simulink model "am_ssb_moding_sine_signal"  (R2022b)
settings: Solver=VariableStepAuto  StartTime=0.0  StopTime=0.06  RelTol=1e-3
undefined symbols (not defined in the file or in its folder): fdesignblkfcn, gcbh
libraries: dspsrcs4 x6
settings Model: Creator=kalyan  LastModifiedBy=kalyan

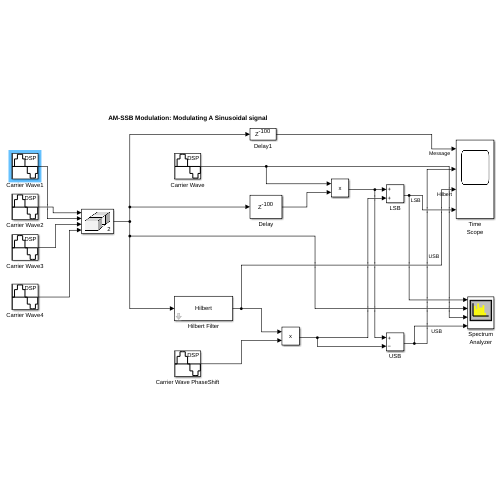
[thumbnail: Simulink's stored preview of the top-level diagram]
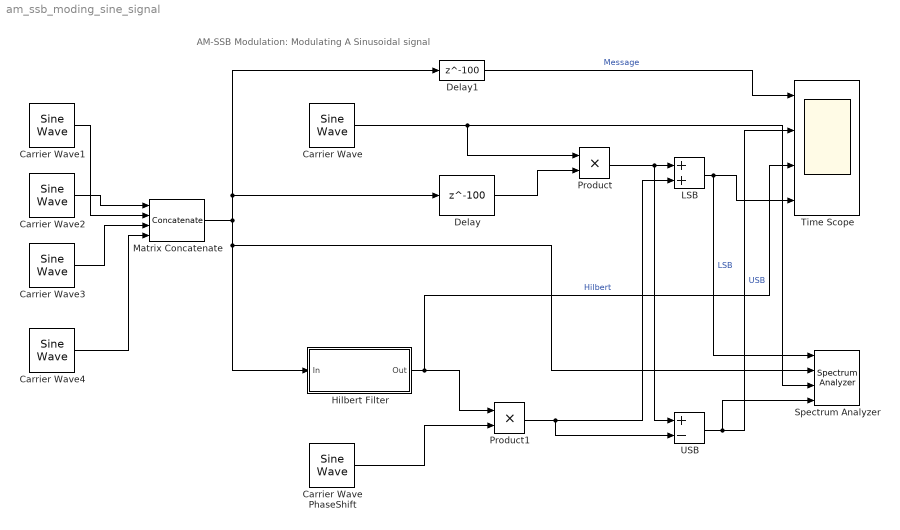
== system am_ssb_moding_sine_signal ==
  note: AM-SSB Modulation: Modulating A Sinusoidal signal
  Carrier Wave{,1..4} (5 alike) : dspsrcs4/Sine Wave  Amplitude=3  Frequency=15000  Phase=1.5708  SampleMode=Discrete  OutComplex=Real  CompMethod=Trigonometric fcn  TableSize=Speed  SampleTime=1/200000  SamplesPerFrame=1  ResetState=Restart at time zero  OutputFrames=off  dataType=double  wordLen=16  udDataType=sfix(16)  fracBitsMode=Best precision  numFracBits=15  OutDataTypeStr=double  LastOutDataTypeStr=double
  Carrier Wave PhaseShift : dspsrcs4/Sine Wave  Amplitude=3  Frequency=15000  Phase=1.5708 - (pi/2)  SampleMode=Discrete  OutComplex=Real  CompMethod=Trigonometric fcn  TableSize=Speed  SampleTime=1/200000  SamplesPerFrame=1  ResetState=Restart at time zero  OutputFrames=off  dataType=double  wordLen=16  udDataType=sfix(16)  fracBitsMode=Best precision  numFracBits=15  OutDataTypeStr=double  LastOutDataTypeStr=double
  Delay : Delay  DelayLength=100  InitialCondition=0  UseCircularBuffer=on
  Delay1 : Delay  DelayLength=100  InitialCondition=0  UseCircularBuffer=on
  Hilbert Filter : Subsystem  DialogController=fdesignblkfcn  InitFcn=fdesignblkfcn(gcbh, {'InitFcn'});  mask(Hilbert Filter){}
      mask help: Design a Hilbert filter
      settings: CopyFcn=fdesignblkfcn(gcbh, {'CopyFcn'});
      mask Help: helpview(mapfilelocation('dsp'), 'dsphilbertfilter');
      mask Display: disp('Hilbert')
  LSB : Sum
  Matrix Concatenate : Concatenate  NumInputs=4  Mode=Multidimensional array  ConcatenateDimension=2
  Product : Product
  Product1 : Product
  Spectrum Analyzer : SpectrumAnalyzer  NumInputPorts=4
  Time Scope : Scope  NumInputPorts=4
  USB : Sum  Inputs=+-
  wires:
  Matrix Concatenate/1 -> Spectrum Analyzer/2, Hilbert Filter/1(In), Delay1/1, Delay/1
  Delay/1 -> Product/2
  Carrier Wave/1 -> Spectrum Analyzer/3, Product/1
  Carrier Wave PhaseShift/1 -> Product1/2
  Hilbert Filter/1(Out) -> Time Scope/3, Product1/1  "Hilbert"
  Product/1 -> USB/1, LSB/1
  Product1/1 -> USB/2, LSB/2
  LSB/1 -> Spectrum Analyzer/1, Time Scope/4  "LSB"
  USB/1 -> Spectrum Analyzer/4, Time Scope/2  "USB"
  Delay1/1 -> Time Scope/1  "Message"
  Carrier Wave1/1 -> Matrix Concatenate/2
  Carrier Wave2/1 -> Matrix Concatenate/1
  Carrier Wave3/1 -> Matrix Concatenate/3
  Carrier Wave4/1 -> Matrix Concatenate/4

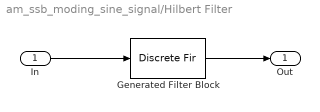
== system am_ssb_moding_sine_signal/Hilbert Filter ==
  In : Inport
  Generated Filter Block : DiscreteFir  Tag=BlockMethodSubSystem  Coefficients=[5.15003860718366009e-16 -8.3766156093727947e-05 2.35802139276509804e-15 -6.59921120241440854e-05 -6.21131926040260173e-16 -9.1525954819813264e-05 -2.00176151456124911e-15 -0.000123132434560440258 -3.05107280552708726e-16 -0.000161730665024954116 1.75952430435556519e-16 -0.000208423670586796493 2.01587097254586396e-15 -0.000264383211643709698 -1.610281707376286e-15 -0.000330710011787250114 4.47980881876914342e-16 -0.000408696011035433043 4.0072562979169073e-16 -0.000499931565631960007 6.30207115560208947e-18 -0.00060563845625784523 -1.85182186360100157e-15 -0.000727692106649796902 4.58452752684780493e-16 -0.000867679981296772679 -9.76830925643750307e-16 -0.00102747560730318162 4.09443805471711121e-17 -0.00120901537620928673 -1.12671199314682863e-15 -0.00141440718247402494 1.05728971394581867e-16 -0.00164584721433578759 -1.09123485116408545e-15 -0.00190572821198673609 -6.15070880281911073e-17 -0.00219664594566571642 -2.63235531544125575e-15 -0.00252127208500864397 -9.86220006547336938e-17 -0.00288263170640534749 -2.23155877222714893e-15 -0.00328388821373934436 6.80564448034878998e-16 -0.00372856932795255502 -2.2104513355667737e-15 -0.00422052960674552946 -2.88101162274187891e-15 -0.0047640841311787363 -4.46878665199657658e-16 -0.00536402966998528186 -1.42657281881564379e-15 -0.0060258227885991722 -1.99609070197495857e-15 -0.00675570742237388555 -1.64783816043889293e-15 -0.0075608679903074183 -3.44945667225607795e-15 -0.00844978651450961626 -5.51511027392387909e-16 -0.00943247240120809183 -1.65974204253792809e-15 -0.0105210003688205878 -2.95985059738225901e-15 -0.0117300539603795717 -2.39566240661592351e-15 -0.0130778024929272263 -1.12147932381843187e-15 -0.0145869975917447547 -2.06491288782388946e-15 -0.0162866548954166968 -1.81693710203142217e-15 -0.0182143841781513549 -1.65833976762791743e-15 -0.0204198729628535247 -1.84779194984796564e-15 -0.0229702377201820296 -1.8845422584866619e-15 -0.0259583148116095952 -1.85614522192180486e-15 -0.0295163237229347786 -3.19112514843393867e-16 -0.0338390396560239726 -2.72936028724128852e-15 -0.0392256295243038622 -3.25732703759293152e-16 -0.0461599683542128769 -1.84723877335595613e-15 -0.0554787131857730209 -6.95726387337531953e-17 -0.0687633279679844556 -1.2271166009295242e-15 -0.0894042367244471947 -5.82444727541570988e-16 -0.126218882474189442 -4.54828504509317286e-16 -0.211541923687201816 -2.46950975548743894e-16 -0.636397947780191764 0 0.636397947780191764 2.46950975548743894e-16 0.211541923687201816 4.54828504509317286e-16 0.126218882474189442 5.82444727541570988e-16 0.0894042367244471947 1.2271166009295242e-15 0.0687633279679844556 6.95726387337531953e-17 0.0554787131857730209 1.84723877335595613e-15 0.0461599683542128769 3.25732703759293152e-16 0.0392256295243038622 2.72936028724128852e-15 0.0338390396560239726 3.19112514843393867e-16 0.0295163237229347786 1.85614522192180486e-15 0.0259583148116095952 1.8845422584866619e-15 0.0229702377201820296 1.84779194984796564e-15 0.0204198729628535247 1.65833976762791743e-15 0.0182143841781513549 1.81693710203142217e-15 0.0162866548954166968 2.06491288782388946e-15 0.0145869975917447547 1.12147932381843187e-15 0.0130778024929272263 2.39566240661592351e-15 0.0117300539603795717 2.95985059738225901e-15 0.0105210003688205878 1.65974204253792809e-15 0.00943247240120809183 5.51511027392387909e-16 0.00844978651450961626 3.44945667225607795e-15 0.0075608679903074183 1.64783816043889293e-15 0.00675570742237388555 1.99609070197495857e-15 0.0060258227885991722 1.42657281881564379e-15 0.00536402966998528186 4.46878665199657658e-16 0.0047640841311787363 2.88101162274187891e-15 0.00422052960674552946 2.2104513355667737e-15 0.00372856932795255502 -6.80564448034878998e-16 0.00328388821373934436 2.23155877222714893e-15 0.00288263170640534749 9.86220006547336938e-17 0.00252127208500864397 2.63235531544125575e-15 0.00219664594566571642 6.15070880281911073e-17 0.00190572821198673609 1.09123485116408545e-15 0.00164584721433578759 -1.05728971394581867e-16 ...(+768 chars)]
  Out : Outport  VectorParamsAs1DForOutWhenUnconnected=off
  wires:
  Generated Filter Block/1 -> Out/1
  In/1 -> Generated Filter Block/1
